simulink subsystem "Push_button_to_Toggle_Switch"  (R2023a)
settings: Solver=VariableStepAuto  StartTime=0.0  StopTime=10.0  RelTol=1e-3
libraries: dspsigops x1
settings Model: Creator=gcs_comp1  LastModifiedBy=gcs_comp1

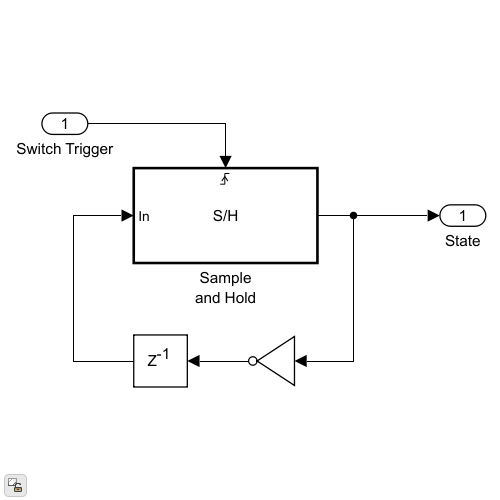
[thumbnail: Simulink's stored preview of the top-level diagram]
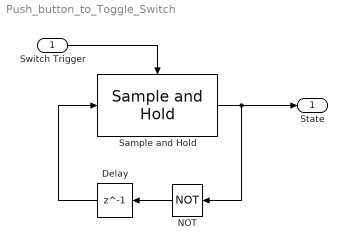
== system Push_button_to_Toggle_Switch ==
  Switch Trigger : Inport
  Delay : Delay  DelayLength=1  InitialCondition=false
  NOT : Logic  Operator=NOT  IconShape=distinctive  AllPortsSameDT=off  OutDataTypeStr=boolean
  Sample and Hold : dspsigops/Sample and Hold  trig=Rising edge  initCond=false  latchinput=off
  State : Outport
  wires:
  Sample and Hold/1 -> NOT/1, State/1
  NOT/1 -> Delay/1
  Delay/1 -> Sample and Hold/1
  Switch Trigger/1 -> Sample and Hold/Trigger
